simulink model "v13_D_flipflops"  (R2019b)
settings: Solver=FixedStepAuto  StartTime=0.0  StopTime=inf  FixedStep=1  MaxStep=1  RelTol=1e-3
libraries: simulink_extras x1
settings Model: NumberOfSteps=2  Creator=MARAT  LastModifiedBy=Marat
settings SFSimCC: CustomCodeUndefinedFunction=UseInterfaceOnly

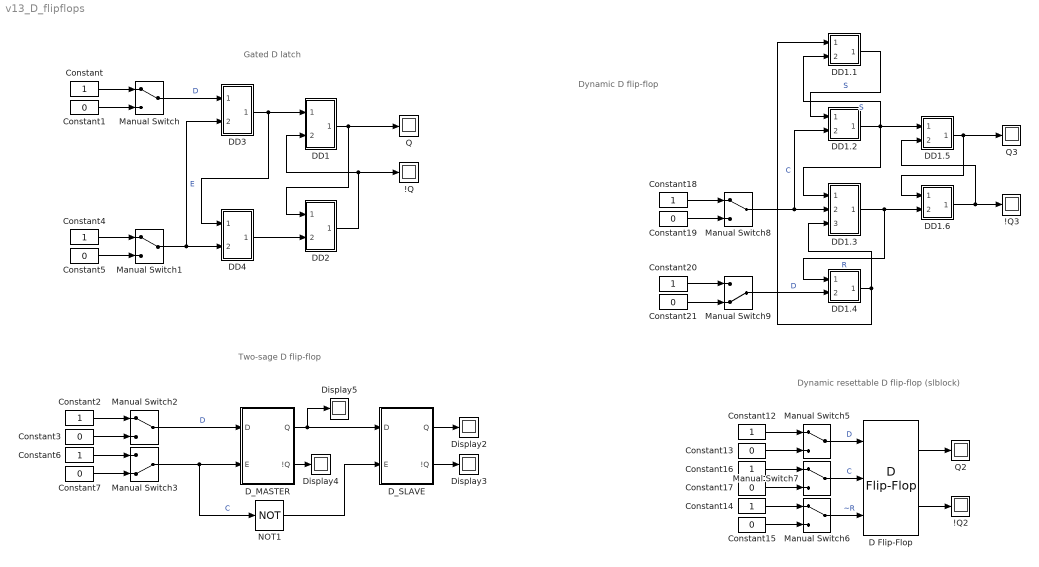
== system v13_D_flipflops ==
  note: Gated D latch
  note: Two-sage D flip-flop
  note: Dynamic D flip-flop
  note: Dynamic resettable D flip-flop (slblock)
  !Q : Display
  !Q2 : Display
  !Q3 : Display
  Constant{,2,4,6,12,14,16,18,20} (9 alike) : Constant  OutDataTypeStr=boolean
  Constant{1,3,5,7,13,15,17,19,21} (9 alike) : Constant  Value=0  OutDataTypeStr=boolean
  D Flip-Flop : simulink_extras/Flip Flops/D Flip-Flop
      settings: SourceProductName=Simulink
  DD1 : Subsystem
      mask Display: disp('&~');
  DD1.1 : Subsystem
      mask Display: disp('&~');
  DD1.2 : Subsystem
      mask Display: disp('&~');
  DD1.3 : Subsystem
      mask Display: disp('&~');
  DD1.4 : Subsystem
      mask Display: disp('&~');
  DD1.5 : Subsystem
      mask Display: disp('&~');
  DD1.6 : Subsystem
      mask Display: disp('&~');
  DD2 : Subsystem
      mask Display: disp('&~');
  DD3 : Subsystem
      mask Display: disp('&~');
  DD4 : Subsystem
      mask Display: disp('&~');
  D_MASTER : Subsystem
  D_SLAVE : Subsystem
  Display{2..5} (4 alike) : Display
  Manual Switch{,1..2,5..8} (7 alike) : ManualSwitch
  Manual Switch3 : ManualSwitch  CurrentSetting=0
  Manual Switch9 : ManualSwitch  CurrentSetting=0
  NOT1 : Logic  Operator=NOT  IconShape=distinctive  AllPortsSameDT=off  OutDataTypeStr=boolean
  Q : Display
  Q2 : Display
  Q3 : Display
  wires:
  Constant1/1 -> Manual Switch/2
  Constant/1 -> Manual Switch/1
  Constant5/1 -> Manual Switch1/2
  Constant4/1 -> Manual Switch1/1
  Manual Switch/1 -> DD3/1(In1)  "D"
  Manual Switch1/1 -> DD3/2(In2), DD4/2(In2)  "E"
  DD1/1(Out1) -> Q/1, DD2/1(In1)
  DD2/1(Out1) -> DD1/2(In2), !Q/1
  DD3/1(Out1) -> DD4/1(In1), DD1/1(In1)
  DD4/1(Out1) -> DD2/2(In2)
  Constant6/1 -> Manual Switch3/1
  NOT1/1 -> D_SLAVE/2(E)
  Constant7/1 -> Manual Switch3/2
  Manual Switch3/1 -> D_MASTER/2(E), NOT1/1  "C"
  D_MASTER/1(Q) -> Display5/1, D_SLAVE/1(D)
  D_MASTER/2(!Q) -> Display4/1
  D_SLAVE/1(Q) -> Display2/1
  Manual Switch2/1 -> D_MASTER/1(D)  "D"
  D_SLAVE/2(!Q) -> Display3/1
  Constant3/1 -> Manual Switch2/2
  Constant2/1 -> Manual Switch2/1
  Constant13/1 -> Manual Switch5/2
  Constant14/1 -> Manual Switch6/1
  Constant12/1 -> Manual Switch5/1
  Constant15/1 -> Manual Switch6/2
  Manual Switch6/1 -> D Flip-Flop/3  "~R"
  Constant16/1 -> Manual Switch7/1
  Constant17/1 -> Manual Switch7/2
  Manual Switch7/1 -> D Flip-Flop/2  "C"
  Manual Switch5/1 -> D Flip-Flop/1  "D"
  D Flip-Flop/1 -> Q2/1
  D Flip-Flop/2 -> !Q2/1
  Constant19/1 -> Manual Switch8/2
  Manual Switch9/1 -> DD1.4/2(In2)  "D"
  Constant20/1 -> Manual Switch9/1
  Constant18/1 -> Manual Switch8/1
  Manual Switch8/1 -> DD1.3/2(In2), DD1.2/2(In2)  "C"
  Constant21/1 -> Manual Switch9/2
  DD1.5/1(Out1) -> Q3/1, DD1.6/1(In1)
  DD1.6/1(Out1) -> !Q3/1, DD1.5/2(In2)
  DD1.2/1(Out1) -> DD1.1/2(In2), DD1.3/1(In1), DD1.5/1(In1)  "S"
  DD1.3/1(Out1) -> DD1.4/1(In1), DD1.6/2(In2)  "R"
  DD1.4/1(Out1) -> DD1.3/3(In3), DD1.1/1(In1)
  DD1.1/1(Out1) -> DD1.2/1(In1)  "S"

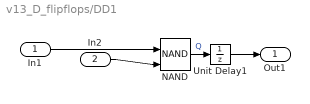
== system v13_D_flipflops/DD1 ==
  In1 : Inport
  In2 : Inport  Port=2
  NAND : Logic  Operator=NAND  IconShape=distinctive  AllPortsSameDT=off  OutDataTypeStr=boolean
  Unit Delay1 : UnitDelay  SampleTime=-1  HasFrameUpgradeWarning=on
  Out1 : Outport
  wires:
  NAND/1 -> Unit Delay1/1  "Q"
  Unit Delay1/1 -> Out1/1
  In1/1 -> NAND/1
  In2/1 -> NAND/2

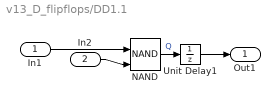
== system v13_D_flipflops/DD1.1 ==
  In1 : Inport
  In2 : Inport  Port=2
  NAND : Logic  Operator=NAND  IconShape=distinctive  AllPortsSameDT=off  OutDataTypeStr=boolean
  Unit Delay1 : UnitDelay  SampleTime=-1  HasFrameUpgradeWarning=on
  Out1 : Outport
  wires:
  In2/1 -> NAND/2
  In1/1 -> NAND/1
  Unit Delay1/1 -> Out1/1
  NAND/1 -> Unit Delay1/1  "Q"

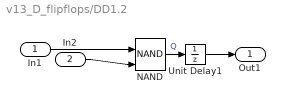
== system v13_D_flipflops/DD1.2 ==
  In1 : Inport
  In2 : Inport  Port=2
  NAND : Logic  Operator=NAND  IconShape=distinctive  AllPortsSameDT=off  OutDataTypeStr=boolean
  Unit Delay1 : UnitDelay  SampleTime=-1  HasFrameUpgradeWarning=on
  Out1 : Outport
  wires:
  NAND/1 -> Unit Delay1/1  "Q"
  Unit Delay1/1 -> Out1/1
  In1/1 -> NAND/1
  In2/1 -> NAND/2

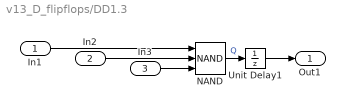
== system v13_D_flipflops/DD1.3 ==
  In1 : Inport
  In2 : Inport  Port=2
  In3 : Inport  Port=3
  NAND : Logic  Operator=NAND  Inputs=3  IconShape=distinctive  AllPortsSameDT=off  OutDataTypeStr=boolean
  Unit Delay1 : UnitDelay  SampleTime=-1  HasFrameUpgradeWarning=on
  Out1 : Outport
  wires:
  In3/1 -> NAND/3
  In2/1 -> NAND/2
  In1/1 -> NAND/1
  Unit Delay1/1 -> Out1/1
  NAND/1 -> Unit Delay1/1  "Q"

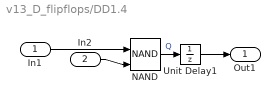
== system v13_D_flipflops/DD1.4 ==
  In1 : Inport
  In2 : Inport  Port=2
  NAND : Logic  Operator=NAND  IconShape=distinctive  AllPortsSameDT=off  OutDataTypeStr=boolean
  Unit Delay1 : UnitDelay  SampleTime=-1  HasFrameUpgradeWarning=on
  Out1 : Outport
  wires:
  In2/1 -> NAND/2
  In1/1 -> NAND/1
  Unit Delay1/1 -> Out1/1
  NAND/1 -> Unit Delay1/1  "Q"

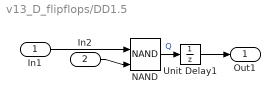
== system v13_D_flipflops/DD1.5 ==
  In1 : Inport
  In2 : Inport  Port=2
  NAND : Logic  Operator=NAND  IconShape=distinctive  AllPortsSameDT=off  OutDataTypeStr=boolean
  Unit Delay1 : UnitDelay  SampleTime=-1  HasFrameUpgradeWarning=on
  Out1 : Outport
  wires:
  NAND/1 -> Unit Delay1/1  "Q"
  Unit Delay1/1 -> Out1/1
  In1/1 -> NAND/1
  In2/1 -> NAND/2

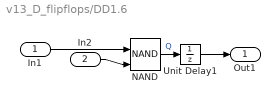
== system v13_D_flipflops/DD1.6 ==
  In1 : Inport
  In2 : Inport  Port=2
  NAND : Logic  Operator=NAND  IconShape=distinctive  AllPortsSameDT=off  OutDataTypeStr=boolean
  Unit Delay1 : UnitDelay  SampleTime=-1  HasFrameUpgradeWarning=on
  Out1 : Outport
  wires:
  In2/1 -> NAND/2
  In1/1 -> NAND/1
  Unit Delay1/1 -> Out1/1
  NAND/1 -> Unit Delay1/1  "Q"

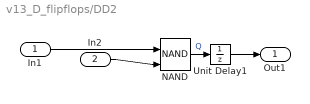
== system v13_D_flipflops/DD2 ==
  In1 : Inport
  In2 : Inport  Port=2
  NAND : Logic  Operator=NAND  IconShape=distinctive  AllPortsSameDT=off  OutDataTypeStr=boolean
  Unit Delay1 : UnitDelay  SampleTime=-1  HasFrameUpgradeWarning=on
  Out1 : Outport
  wires:
  In2/1 -> NAND/2
  In1/1 -> NAND/1
  Unit Delay1/1 -> Out1/1
  NAND/1 -> Unit Delay1/1  "Q"

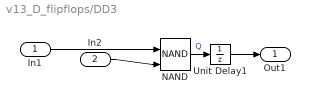
== system v13_D_flipflops/DD3 ==
  In1 : Inport
  In2 : Inport  Port=2
  NAND : Logic  Operator=NAND  IconShape=distinctive  AllPortsSameDT=off  OutDataTypeStr=boolean
  Unit Delay1 : UnitDelay  SampleTime=-1  HasFrameUpgradeWarning=on
  Out1 : Outport
  wires:
  In2/1 -> NAND/2
  In1/1 -> NAND/1
  Unit Delay1/1 -> Out1/1
  NAND/1 -> Unit Delay1/1  "Q"

== system v13_D_flipflops/DD4 ==
  In1 : Inport
  In2 : Inport  Port=2
  NAND : Logic  Operator=NAND  IconShape=distinctive  AllPortsSameDT=off  OutDataTypeStr=boolean
  Unit Delay1 : UnitDelay  SampleTime=-1  HasFrameUpgradeWarning=on
  Out1 : Outport
  wires:
  NAND/1 -> Unit Delay1/1  "Q"
  Unit Delay1/1 -> Out1/1
  In1/1 -> NAND/1
  In2/1 -> NAND/2

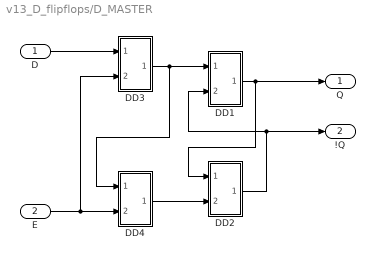
== system v13_D_flipflops/D_MASTER ==
  D : Inport
  E : Inport  Port=2
  DD1 : Subsystem
      mask Display: disp('&~');
  DD2 : Subsystem
      mask Display: disp('&~');
  DD3 : Subsystem
      mask Display: disp('&~');
  DD4 : Subsystem
      mask Display: disp('&~');
  Q : Outport
  !Q : Outport  Port=2
  wires:
  DD3/1(Out1) -> DD4/1(In1), DD1/1(In1)
  DD1/1(Out1) -> Q/1, DD2/1(In1)
  DD2/1(Out1) -> !Q/1, DD1/2(In2)
  E/1 -> DD3/2(In2), DD4/2(In2)
  DD4/1(Out1) -> DD2/2(In2)
  D/1 -> DD3/1(In1)

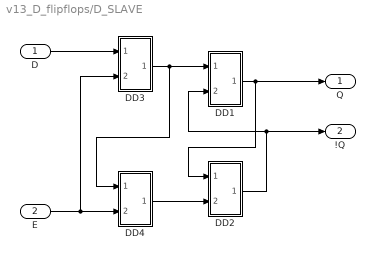
== system v13_D_flipflops/D_SLAVE ==
  D : Inport
  E : Inport  Port=2
  DD1 : Subsystem
      mask Display: disp('&~');
  DD2 : Subsystem
      mask Display: disp('&~');
  DD3 : Subsystem
      mask Display: disp('&~');
  DD4 : Subsystem
      mask Display: disp('&~');
  Q : Outport
  !Q : Outport  Port=2
  wires:
  D/1 -> DD3/1(In1)
  DD4/1(Out1) -> DD2/2(In2)
  E/1 -> DD4/2(In2), DD3/2(In2)
  DD2/1(Out1) -> DD1/2(In2), !Q/1
  DD1/1(Out1) -> DD2/1(In1), Q/1
  DD3/1(Out1) -> DD1/1(In1), DD4/1(In1)

== system v13_D_flipflops/D_MASTER/DD1 ==
  In1 : Inport
  In2 : Inport  Port=2
  NAND : Logic  Operator=NAND  IconShape=distinctive  AllPortsSameDT=off  OutDataTypeStr=boolean
  Unit Delay1 : UnitDelay  SampleTime=-1  HasFrameUpgradeWarning=on
  Out1 : Outport
  wires:
  NAND/1 -> Unit Delay1/1  "Q"
  Unit Delay1/1 -> Out1/1
  In1/1 -> NAND/1
  In2/1 -> NAND/2

== system v13_D_flipflops/D_MASTER/DD2 ==
  In1 : Inport
  In2 : Inport  Port=2
  NAND : Logic  Operator=NAND  IconShape=distinctive  AllPortsSameDT=off  OutDataTypeStr=boolean
  Unit Delay1 : UnitDelay  SampleTime=-1  HasFrameUpgradeWarning=on
  Out1 : Outport
  wires:
  In2/1 -> NAND/2
  In1/1 -> NAND/1
  Unit Delay1/1 -> Out1/1
  NAND/1 -> Unit Delay1/1  "Q"

== system v13_D_flipflops/D_MASTER/DD3 ==
  In1 : Inport
  In2 : Inport  Port=2
  NAND : Logic  Operator=NAND  IconShape=distinctive  AllPortsSameDT=off  OutDataTypeStr=boolean
  Unit Delay1 : UnitDelay  SampleTime=-1  HasFrameUpgradeWarning=on
  Out1 : Outport
  wires:
  In2/1 -> NAND/2
  In1/1 -> NAND/1
  Unit Delay1/1 -> Out1/1
  NAND/1 -> Unit Delay1/1  "Q"

== system v13_D_flipflops/D_MASTER/DD4 ==
  In1 : Inport
  In2 : Inport  Port=2
  NAND : Logic  Operator=NAND  IconShape=distinctive  AllPortsSameDT=off  OutDataTypeStr=boolean
  Unit Delay1 : UnitDelay  SampleTime=-1  HasFrameUpgradeWarning=on
  Out1 : Outport
  wires:
  NAND/1 -> Unit Delay1/1  "Q"
  Unit Delay1/1 -> Out1/1
  In1/1 -> NAND/1
  In2/1 -> NAND/2

== system v13_D_flipflops/D_SLAVE/DD1 ==
  In1 : Inport
  In2 : Inport  Port=2
  NAND : Logic  Operator=NAND  IconShape=distinctive  AllPortsSameDT=off  OutDataTypeStr=boolean
  Unit Delay1 : UnitDelay  SampleTime=-1  HasFrameUpgradeWarning=on
  Out1 : Outport
  wires:
  In2/1 -> NAND/2
  In1/1 -> NAND/1
  Unit Delay1/1 -> Out1/1
  NAND/1 -> Unit Delay1/1  "Q"

== system v13_D_flipflops/D_SLAVE/DD2 ==
  In1 : Inport
  In2 : Inport  Port=2
  NAND : Logic  Operator=NAND  IconShape=distinctive  AllPortsSameDT=off  OutDataTypeStr=boolean
  Unit Delay1 : UnitDelay  SampleTime=-1  HasFrameUpgradeWarning=on
  Out1 : Outport
  wires:
  NAND/1 -> Unit Delay1/1  "Q"
  Unit Delay1/1 -> Out1/1
  In1/1 -> NAND/1
  In2/1 -> NAND/2

== system v13_D_flipflops/D_SLAVE/DD3 ==
  In1 : Inport
  In2 : Inport  Port=2
  NAND : Logic  Operator=NAND  IconShape=distinctive  AllPortsSameDT=off  OutDataTypeStr=boolean
  Unit Delay1 : UnitDelay  SampleTime=-1  HasFrameUpgradeWarning=on
  Out1 : Outport
  wires:
  NAND/1 -> Unit Delay1/1  "Q"
  Unit Delay1/1 -> Out1/1
  In1/1 -> NAND/1
  In2/1 -> NAND/2

== system v13_D_flipflops/D_SLAVE/DD4 ==
  In1 : Inport
  In2 : Inport  Port=2
  NAND : Logic  Operator=NAND  IconShape=distinctive  AllPortsSameDT=off  OutDataTypeStr=boolean
  Unit Delay1 : UnitDelay  SampleTime=-1  HasFrameUpgradeWarning=on
  Out1 : Outport
  wires:
  In2/1 -> NAND/2
  In1/1 -> NAND/1
  Unit Delay1/1 -> Out1/1
  NAND/1 -> Unit Delay1/1  "Q"
